simulink model "pneumaticmodelwithpressuredynamic"  (R2013a)
settings: Solver=ode4  StartTime=0.0  StopTime=20  FixedStep=0.005  RelTol=1e-3
libraries: simulink x5, cstblocks x5
settings Model: Creator=gkharish  LastModifiedBy=gkharish

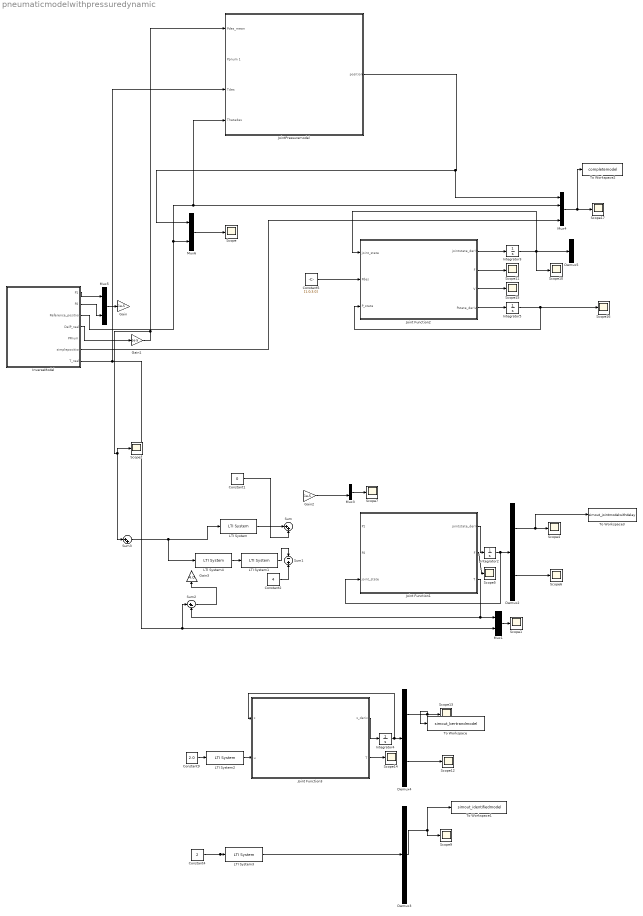
== system pneumaticmodelwithpressuredynamic ==
  Constant1 : Constant  Value=0
  Constant2 : Constant  Value=4
  Constant4 : Constant  Value=2
  Constant5 : Constant  Value=[1.0;3.0]
  Constant9 : Constant  Value=2.0
  Demux2 : Demux  Outputs=2
  Demux3 : Demux  Outputs=1
  Demux4 : Demux  Outputs=2
  Demux5 : Demux  Outputs=2
  Gain : Gain  Gain=1e-5
  Gain1 : Gain  Gain=1e-5
  Gain2 : Gain  Gain=1e-5
  Gain3 : Gain  Gain=4.0
  Integrator2 : Integrator  InitialCondition=[0 0]
  Integrator3 : Integrator  InitialCondition=[0 0]
  Integrator4 : Integrator  InitialCondition=[0 0]
  Integrator5 : Integrator  InitialCondition=[0 0 4 0]
  InverseModel : Subsystem
  Joint Function1 : MATLAB Function  TreatAsAtomicUnit=on
  Joint Function2 : MATLAB Function  TreatAsAtomicUnit=on
  Joint Function3 : MATLAB Function  TreatAsAtomicUnit=on
  "JointPressuremodel " : Subsystem
  LTI System : cstblocks/LTI System  sys=tf(1, [0.17 1])  IC=[]
  LTI System1 : cstblocks/LTI System  sys=tf(1, [0.5 1])  IC=[]
  LTI System2 : cstblocks/LTI System  sys=tf(1, [0.2 1])  IC=[]
  LTI System3 : cstblocks/LTI System  sys=tf(1, [0.17 1])  IC=[]
  LTI System4 : cstblocks/LTI System  sys=tf(1, [0.5 1])  IC=[]
  Mux1 : Mux  Inputs=2
  Mux3 : Mux  Inputs=3
  Mux4 : Mux
  Mux5 : Mux  Inputs=2
  Mux6 : Mux  Inputs=2
  Scope{,1..2,4..7,9..17} (16 alike) : Scope
      Scope settings: SaveName=ScopeData19
      Scope1 settings: ShowLegends=on  SaveName=ScopeData26
      Scope10 settings: SaveName=ScopeData9
      Scope11 settings: SaveName=ScopeData11
      Scope12 settings: SaveName=ScopeData12
      Scope13 settings: ShowLegends=on  SaveName=ScopeData13
      Scope14 settings: ShowLegends=on  SaveName=ScopeData14
      Scope15 settings: ShowLegends=on  SaveName=ScopeData15
      Scope16 settings: SaveName=ScopeData16
      Scope17 settings: ShowLegends=on  YMin=-0.8  YMax=0.9  SaveName=ScopeData17
      Scope2 settings: ShowLegends=on  SaveName=ScopeData28
      Scope4 settings: ShowLegends=on  SaveName=ScopeData4
      Scope5 settings: ShowLegends=on  SaveName=ScopeData5
      Scope6 settings: SaveName=ScopeData6
      Scope7 settings: ShowLegends=on  SaveName=ScopeData7
      Scope9 settings: ShowLegends=on  SaveName=ScopeData10
  Sum : Sum  Inputs=|++
  Sum1 : Sum  Inputs=-+
  Sum2 : Sum  Inputs=|+-
  Sum3 : Sum  Inputs=|++
  To Workspace : ToWorkspace  VariableName=simout_bertrandmodel  SampleTime=-1  SaveFormat=Timeseries
  To Workspace1 : ToWorkspace  VariableName=simout_identifiedmodel  SampleTime=-1  SaveFormat=Timeseries
  To Workspace2 : ToWorkspace  VariableName=completemodel  SampleTime=-1  SaveFormat=Timeseries
  To Workspace3 : ToWorkspace  VariableName=simout_jointmodelwithdelay  SampleTime=-1  SaveFormat=Timeseries
  wires:
  Joint Function1/1(jointstate_deriv) -> Integrator2/1
  Integrator2/1 -> Demux2/1, Joint Function1/3(joint_state)
  Demux2/1 -> To Workspace3/1, Scope4/1
  Joint Function1/2(F) -> Scope5/1
  Demux2/2 -> Scope6/1
  Mux3/1 -> Scope7/1
  InverseModel/4(DelP_real) -> Gain1/1
  Joint Function3/1(x_deriv) -> Integrator4/1
  Integrator4/1 -> Joint Function3/1(x), Demux4/1
  Demux4/1 -> To Workspace/1, Scope13/1
  Demux4/2 -> Scope12/1
  Joint Function3/2(T) -> Scope14/1
  Demux3/1 -> Scope9/1, To Workspace1/1
  LTI System3/1 -> Demux3/1
  Constant4/1 -> LTI System3/1
  Joint Function2/1(jointstate_deriv) -> Integrator3/1
  Joint Function2/4(Pstate_deriv) -> Integrator5/1
  Integrator3/1 -> Scope10/1, Demux5/1, Joint Function2/1(joint_state)
  Joint Function2/2(F) -> Scope11/1
  Joint Function2/3(V) -> Scope15/1
  Integrator5/1 -> Joint Function2/3(P_state), Scope16/1
  Constant5/1 -> Joint Function2/2(Pdes)
  Mux4/1 -> To Workspace2/1, Scope17/1
  Constant9/1 -> LTI System2/1
  LTI System2/1 -> Joint Function3/2(u)
  Mux6/1 -> Scope/1
  Mux5/1 -> Gain/1
  InverseModel/1(P1) -> Mux5/1
  InverseModel/2(P2) -> Mux5/2
  InverseModel/3(Reference_position) -> "JointPressuremodel "/4(Thetades), Mux4/2, Mux6/2
  "JointPressuremodel "/1(position) -> Mux4/1, Mux6/1
  InverseModel/6(simpleposition) -> Mux4/4
  Gain2/1 -> Mux3/3
  Joint Function1/3(T) -> Mux1/1, Sum2/2
  Mux1/1 -> Scope1/1
  InverseModel/7(T_real) -> "JointPressuremodel "/3(Tdes), Sum2/1, Mux1/2
  Sum2/1 -> Gain3/1
  Gain1/1 -> "JointPressuremodel "/1("Pdes_mean "), Scope2/1, Sum3/1
  Sum3/1 -> LTI System/1, LTI System4/1
  Constant2/1 -> Sum1/2
  LTI System1/1 -> Sum1/1
  LTI System/1 -> Sum/1
  Constant1/1 -> Sum/2
  LTI System4/1 -> LTI System1/1
  ? -> Mux4/3

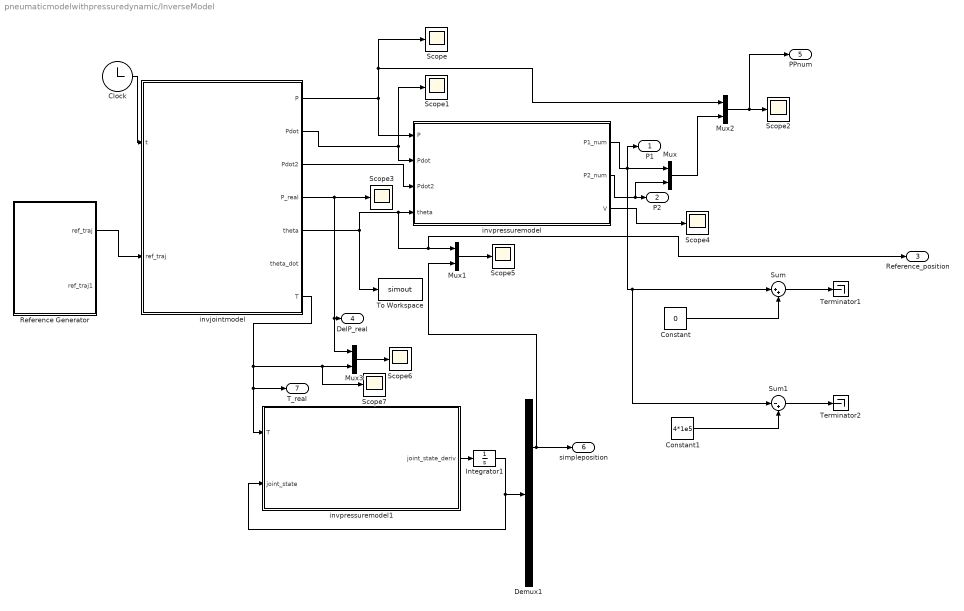
== system pneumaticmodelwithpressuredynamic/InverseModel ==
  Clock : Clock
  Constant : Constant  Value=0
  Constant1 : Constant  Value=4*1e5
  Demux1 : Demux  Outputs=2
  Integrator1 : Integrator  InitialCondition=[0 0]
  Mux{,1..3} (4 alike) : Mux  Inputs=2
  Reference Generator : Subsystem
  Scope{,1..7} (8 alike) : Scope
      Scope settings: SaveName=ScopeData8
      Scope1 settings: SaveName=ScopeData9
      Scope2 settings: ShowLegends=on
      Scope4 settings: SaveName=ScopeData2
      Scope5 settings: ShowLegends=on  SaveName=ScopeData22
      Scope6 settings: ShowLegends=on  SaveName=ScopeData23
      Scope7 settings: ShowLegends=on  SaveName=ScopeData24
  Sum : Sum  Inputs=|++
  Sum1 : Sum  Inputs=|-+
  Terminator1 : Terminator
  Terminator2 : Terminator
  To Workspace : ToWorkspace  VariableName=simout  SampleTime=-1  SaveFormat=Timeseries
  invjointmodel : MATLAB Function  TreatAsAtomicUnit=on
  invpressuremodel : MATLAB Function  TreatAsAtomicUnit=on
  invpressuremodel1 : MATLAB Function  TreatAsAtomicUnit=on
  P1 : Outport
  P2 : Outport  Port=2
  Reference_position : Outport  Port=3
  DelP_real : Outport  Port=4
  PPnum : Outport  Port=5
  simpleposition : Outport  Port=6
  T_real : Outport  Port=7
  wires:
  invjointmodel/2(Pdot) -> invpressuremodel/2(Pdot), Scope1/1
  Clock/1 -> invjointmodel/1(t)
  invpressuremodel/1(P1_num) -> P1/1, Mux/1, Sum/1, Sum1/1
  Constant1/1 -> Sum1/2
  invjointmodel/5(theta) -> Reference_position/1, Mux1/1, invpressuremodel/4(theta), To Workspace/1
  Constant/1 -> Sum/2
  invjointmodel/1(P) -> Mux2/1, Scope/1, invpressuremodel/1(P)
  invjointmodel/3(Pdot2) -> invpressuremodel/3(Pdot2)
  Sum/1 -> Terminator1/1
  Sum1/1 -> Terminator2/1
  invpressuremodel/2(P2_num) -> P2/1, Mux/2
  invjointmodel/4(P_real) -> Mux3/1, DelP_real/1, Scope3/1
  invpressuremodel/3(V) -> Scope4/1
  Integrator1/1 -> invpressuremodel1/2(joint_state), Demux1/1
  invpressuremodel1/1(joint_state_deriv) -> Integrator1/1
  Demux1/1 -> simpleposition/1, Mux1/2
  Mux1/1 -> Scope5/1
  Mux/1 -> Mux2/2
  Mux2/1 -> PPnum/1, Scope2/1
  Mux3/1 -> Scope6/1
  invjointmodel/7(T) -> Scope7/1, Mux3/2, T_real/1, invpressuremodel1/1(T)
  Reference Generator/1(ref_traj) -> invjointmodel/2(ref_traj)

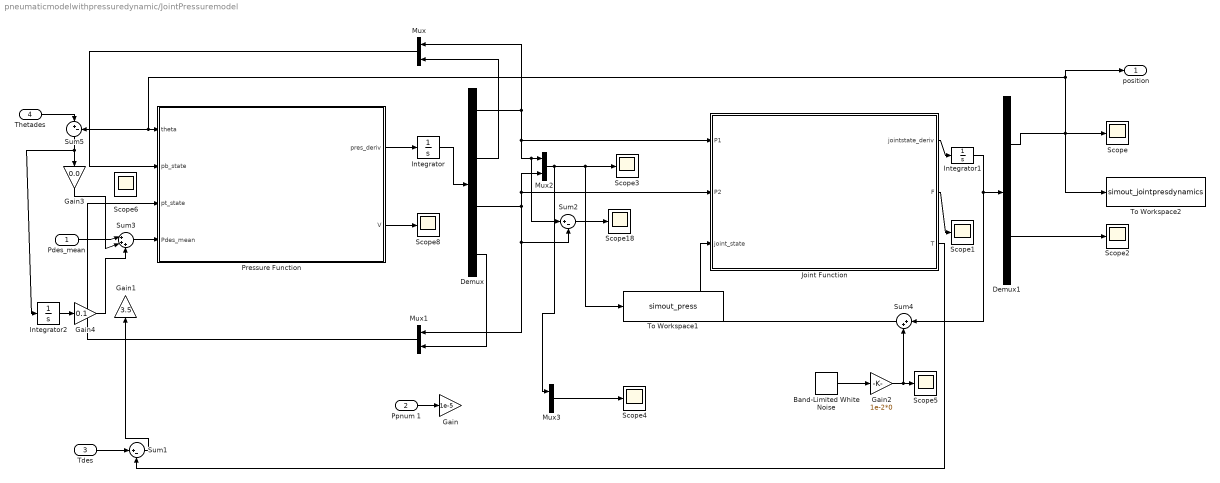
== system pneumaticmodelwithpressuredynamic/JointPressuremodel  ==
  "Pdes_mean " : Inport
  Ppnum 1 : Inport  Port=2
  Tdes : Inport  Port=3
  Thetades : Inport  Port=4
  Band-Limited White Noise : simulink/Sources/Band-Limited White Noise  Cov=[0.1]  Ts=0.005  seed=[23341]
  Demux : Demux
  Demux1 : Demux  Outputs=2
  Gain : Gain  Gain=1e-5
  Gain1 : Gain  Gain=3.5
  Gain2 : Gain  Gain=1e-2*0
  Gain3 : Gain  Gain=0.0
  Gain4 : Gain  Gain=0.1
  Integrator : Integrator  InitialCondition=[0 0 4 0]
  Integrator1 : Integrator  InitialCondition=[0 0]
  Integrator2 : Integrator
  Joint Function : MATLAB Function  TreatAsAtomicUnit=on
  Mux{,1..3} (4 alike) : Mux  Inputs=2
  Pressure Function : MATLAB Function  TreatAsAtomicUnit=on
  Scope{,1..6,8,18} (9 alike) : Scope
      Scope settings: ShowLegends=on
      Scope1 settings: ShowLegends=on  TimeRange=10  YMin=240  YMax=285
      Scope18 settings: ShowLegends=on  SaveName=ScopeData18
      Scope2 settings: SaveName=ScopeData2
      Scope3 settings: ShowLegends=on  SaveName=ScopeData3
      Scope4 settings: ShowLegends=on  SaveName=ScopeData25
      Scope5 settings: ShowLegends=on  SaveName=ScopeData27
      Scope6 settings: ShowLegends=on  SaveName=ScopeData29
      Scope8 settings: ShowLegends=on  SaveName=ScopeData8
  Sum1 : Sum  Inputs=|+-
  Sum2 : Sum  Inputs=|+-
  Sum3 : Sum  Inputs=|+++
  Sum4 : Sum  Inputs=|++
  Sum5 : Sum  Inputs=|+-
  To Workspace1 : ToWorkspace  VariableName=simout_press  SampleTime=-1  SaveFormat=Timeseries
  To Workspace2 : ToWorkspace  VariableName=simout_jointpresdynamics  SampleTime=-1  SaveFormat=Timeseries
  position : Outport
  wires:
  Demux/1 -> Sum2/1, Mux2/1, Joint Function/1(P1), Mux/1
  Integrator1/1 -> Sum4/1, Demux1/1
  Pressure Function/2(V) -> Scope8/1
  Mux1/1 -> Pressure Function/3(pt_state)
  Demux/2 -> Mux/2
  Joint Function/1(jointstate_deriv) -> Integrator1/1
  Demux/4 -> Mux1/2
  Demux1/2 -> Scope2/1
  Demux1/1 -> To Workspace2/1, Sum5/2, Pressure Function/1(theta), position/1, Scope/1
  Joint Function/2(F) -> Scope1/1
  Pressure Function/1(pres_deriv) -> Integrator/1
  Mux/1 -> Pressure Function/2(pb_state)
  Integrator/1 -> Demux/1
  Sum2/1 -> Scope18/1
  Demux/3 -> Sum2/2, Mux1/1, Mux2/2, Joint Function/2(P2)
  Mux3/1 -> Scope4/1
  Ppnum 1/1 -> Gain/1
  "Pdes_mean "/1 -> Sum3/1
  Sum3/1 -> Pressure Function/4(Pdes_mean)
  Sum1/1 -> Gain1/1
  Mux2/1 -> Mux3/1, To Workspace1/1, Scope3/1
  Joint Function/3(T) -> Sum1/2
  Band-Limited White Noise/1 -> Gain2/1
  Sum4/1 -> Joint Function/3(joint_state)
  Gain2/1 -> Sum4/2, Scope5/1
  Tdes/1 -> Sum1/1
  Thetades/1 -> Sum5/1
  Sum5/1 -> Integrator2/1, Gain3/1
  Integrator2/1 -> Gain4/1
  Gain4/1 -> Sum3/3
  Gain3/1 -> Sum3/2

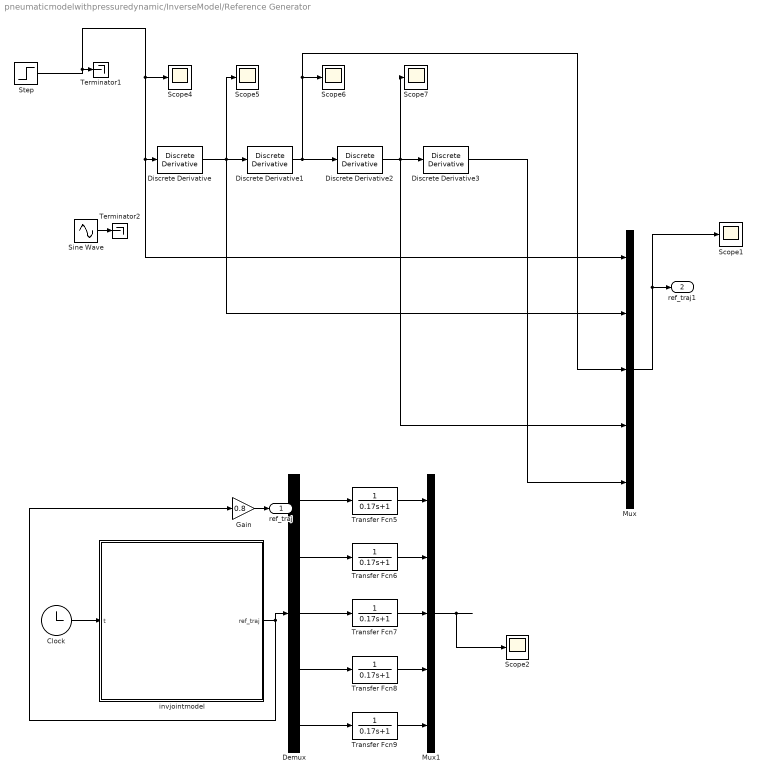
== system pneumaticmodelwithpressuredynamic/InverseModel/Reference Generator ==
  Clock : Clock
  Demux : Demux  Outputs=5
  Discrete Derivative{,1..3} (4 alike) : simulink/Discrete/Discrete Derivative  gainval=1.0  ICPrevScaledInput=0.0  InputProcessing=Inherited  OutMin=[]  OutMax=[]  OutDataType=fixdt(1, 16)  OutScaling=2^-10  DoSatur=off
  Gain : Gain  Gain=0.8
  Mux : Mux  Inputs=5
  Mux1 : Mux  Inputs=5
  Scope{1..2,4..7} (6 alike) : Scope
      Scope1 settings: ShowLegends=on  SaveName=ScopeData20
      Scope2 settings: ShowLegends=on  SaveName=ScopeData21
      Scope4 settings: SaveName=ScopeData4
      Scope5 settings: SaveName=ScopeData5
      Scope6 settings: SaveName=ScopeData6
      Scope7 settings: SaveName=ScopeData7
  Sine Wave : Sin  Amplitude=1.0  SampleTime=0
  Step : Step  SampleTime=0
  Terminator1 : Terminator
  Terminator2 : Terminator
  Transfer Fcn{5..9} (5 alike) : TransferFcn  Denominator=[0.17 1]
  invjointmodel : MATLAB Function  TreatAsAtomicUnit=on
  ref_traj : Outport
  ref_traj1 : Outport  Port=2
  wires:
  Mux/1 -> ref_traj1/1, Scope1/1
  Step/1 -> Mux/1, Discrete Derivative/1, Scope4/1, Terminator1/1
  Discrete Derivative/1 -> Mux/2, Scope5/1, Discrete Derivative1/1
  Discrete Derivative1/1 -> Mux/3, Scope6/1, Discrete Derivative2/1
  Discrete Derivative2/1 -> Mux/4, Discrete Derivative3/1, Scope7/1
  Discrete Derivative3/1 -> Mux/5
  Clock/1 -> invjointmodel/1(t)
  invjointmodel/1(ref_traj) -> Demux/1, Gain/1
  Transfer Fcn5/1 -> Mux1/1
  Transfer Fcn6/1 -> Mux1/2
  Transfer Fcn7/1 -> Mux1/3
  Transfer Fcn8/1 -> Mux1/4
  Transfer Fcn9/1 -> Mux1/5
  Demux/1 -> Transfer Fcn5/1
  Demux/4 -> Transfer Fcn8/1
  Demux/5 -> Transfer Fcn9/1
  Demux/3 -> Transfer Fcn7/1
  Demux/2 -> Transfer Fcn6/1
  Mux1/1 -> Scope2/1
  Gain/1 -> ref_traj/1
  Sine Wave/1 -> Terminator2/1

== matlab function pneumaticmodelwithpressuredynamic/JointPressuremodel /Joint Function ==
  data: P1 input; jointstate_deriv output; P2 input; joint_state input; F output; T output
function [jointstate_deriv,F, T] = jointdynamics(P1, P2, joint_state)
jointstate_deriv = zeros(2,1);
theta = joint_state(1);
theta_dot = joint_state(2);
%% Parameters for the muscles
lo = 0.185;
alphao = 23.0*pi/180;
%epsilono = 0.15;
%emax = 0.2983;
k = 1.25;
ro = 0.009;
R = 0.015;

a = 3/(tan(alphao))^2;
b = 1/(sin(alphao))^2;
emax = (1/k)*(1 - sqrt(b/a));

lb = lo- R*theta;
epsb = (1-(lb/lo));
lt = lo*(1-emax) + R*theta;
epst = (1-(lt/lo));

%% Parameters of Joint
m = 2.6;
link_l = 0.32;
g =9.81;
I = m*(link_l^2)/3;
fv = 0.25;


F1 =  pi*ro^2*P1*1e5*(a*(1-k*epsb)^2 - b);
F2 =  pi*ro^2*P2*1e5*(a*(1-k*epst)^2 - b);
F2max = 1*pi*ro^2*4*1e5*(a*(1-k*emax)^2 - b);
T = (F1 -F2 )*R;
F = [F1 F2 T];
jointstate_deriv(1) = theta_dot; %joint_state(2);
jointstate_deriv(2) = ((F1 -F2 )*R  - fv*theta_dot - m*g*0.5*link_l*sin(theta))/I;

== matlab function pneumaticmodelwithpressuredynamic/JointPressuremodel /Pressure Function ==
  data: theta input; pres_deriv output; pb_state input; pt_state input; Pdes_mean input; V output
function [pres_deriv,V] = pressuredynamics(theta, pb_state, pt_state, Pdes_mean)

pres_deriv = zeros(4,1);
V = zeros(2,1);
Pdes = zeros(2,1);
%% Parameters for the muscles
lo = 0.185;
alphao = 23.0*pi/180;
%epsilono = 0.15;
%emax = 0.2983;
k = 1.25;
ro = 0.009;
R = 0.015;
a = 3/(tan(alphao))^2;
b = 1/(sin(alphao))^2;
emax = (1/k)*(1 - sqrt(b/a));
%% Calculate Volume 
% biceps agonistic muscle
lb = lo - R*theta;
cs2 = (cos(alphao))^2;
epsb2 = (1-(lb/lo))^2;
termb1 = (1 - cs2*epsb2);

Vb = 1e6*(pi*lb*ro^2/((sin(alphao))^2))*termb1
%Vb = 230;
wnb = 2*pi*380*(1/Vb)

% triceps antagonistic muscle 
lt = lo*(1-emax) + R*theta; 
cs2 = (cos(alphao))^2;
epst2 = (1-(lt/lo))^2;
termt1 = (1 - cs2*epst2);

Vt = 1e6*(pi*lt*ro^2/((sin(alphao))^2))*termt1
%Vt = 230;
wnt = 2*pi*380*(1/Vt)

Pdes(1) = Pdes_mean;
Pdes(2) = 4 - Pdes_mean;

pres_deriv(1) = pb_state(2);
pres_deriv(2) = -wnb^2*pb_state(1) - 2*wnb*1*pb_state(2) + (wnb^2)*Pdes(1);

pres_deriv(3) = pt_state(2);
pres_deriv(4) = -wnt^2*pt_state(1) - 2*wnt*1*pt_state(2) + (wnt^2)*Pdes(2);

% pres_deriv(5) = Vb;
% pres_deriv(6) = Vt;
V = [Vb;Vt];

== matlab function pneumaticmodelwithpressuredynamic/Joint Function1 ==
  data: P1 input; jointstate_deriv output; P2 input; joint_state input; F output; T output
function [jointstate_deriv,F,T] = jointdynamics(P1, P2, joint_state)
jointstate_deriv = zeros(2,1);
theta = joint_state(1);
theta_dot = joint_state(2);
%% Parameters for the muscles
lo = 0.185;
alphao = 23.0*pi/180;
%epsilono = 0.15;
%emax = 0.2983;
k = 1.25;
ro = 0.009;
R = 0.015;

a = 3/(tan(alphao))^2;
b = 1/(sin(alphao))^2;
emax = (1/k)*(1 - sqrt(b/a));

lb = lo- R*theta;
epsb = (1-(lb/lo));
lt = lo*(1-emax) + R*theta;
epst = (1-(lt/lo));

%% Parameters of Joint
m = 2.6;
link_l = 0.32;
g =9.81;
I = m*(link_l^2)/3;
fv = 0.25;


F1 =  pi*ro^2*P1*1e5*(a*(1-k*epsb)^2 - b);
F2 =  pi*ro^2*P2*1e5*(a*(1-k*epst)^2 - b);
F2max = 1*pi*ro^2*4*1e5*(a*(1-k*emax)^2 - b);
F = [F1 F2];
jointstate_deriv(1) = theta_dot; %joint_state(2);
jointstate_deriv(2) = ((F1 -F2 )*R  - fv*theta_dot - m*g*0.5*link_l*sin(theta))/I;
T = (F1 -F2 )*R ;

== matlab function pneumaticmodelwithpressuredynamic/Joint Function2 ==
  data: joint_state input; Pdes input; P_state input; jointstate_deriv output; F output; V output; Pstate_deriv output
function [jointstate_deriv,F,V,Pstate_deriv] = jointpressuredynamics(joint_state, Pdes, P_state)
jointstate_deriv = zeros(2,1);
F = zeros(2,1);
V = zeros(2,1);
Pstate_deriv = zeros(4,1);
theta = joint_state(1);
theta_dot = joint_state(2);
%% Parameters for the muscles
lo = 0.185;
alphaob = 23.0*pi/180;
alphaot = 23.0*pi/180;
k = 1.25;
ro = 0.009;
R = 0.015;

a_biceps = 3/(tan(alphaob))^2;
b_biceps = 1/(sin(alphaob))^2;
emax_biceps = (1/k)*(1 - sqrt(b_biceps/a_biceps));

a_triceps = 3/(tan(alphaot))^2;
b_triceps = 1/(sin(alphaot))^2;
emax_triceps = (1/k)*(1 - sqrt(b_triceps/a_triceps));

lb = lo- R*theta;
epsb = (1-(lb/lo));
lt = lo*(1-emax_triceps) + R*theta;
epst = (1-(lt/lo));

%% Parameters of Joint
m = 2.6;
link_l = 0.32;
g =9.81;
I = m*(link_l^2)/3;
fv = 0.25;
%% Volume calcuation
% biceps agonistic muscle
lb = lo - R*theta;
csb2 = (cos(alphaob))^2;
epsb2 = (1-(lb/lo))^2;
termb1 = (1 - csb2*epsb2);

Vb = 1e6*(pi*lb*ro^2/((sin(alphaob))^2))*termb1
%Vb = 1630;
wnb = 2*pi*380*(1/Vb)

% triceps antagonistic muscle 
lt = lo*(1-emax_triceps) + R*theta; 
cst2 = (cos(alphaot))^2;
epst2 = (1-(lt/lo))^2;
termt1 = (1 - cst2*epst2);

Vt = 1e6*(pi*lt*ro^2/((sin(alphaot))^2))*termt1
%Vt = 1630;
wnt = 2*pi*380*(1/Vt)

V = [Vb;Vt];

%% Pressure Dynamics
Pb_state = P_state(1:2,1);
Pt_state = P_state(3:4,1);
Pstate_deriv(1) = Pb_state(2);
Pstate_deriv(2) = -wnb^2*Pb_state(1) - 2*wnb*1*Pb_state(2) + (wnb^2)*Pdes(1);

Pstate_deriv(3) = Pt_state(2);
Pstate_deriv(4) = -wnt^2*Pt_state(1) - 2*wnt*1*Pt_state(2) + (wnt^2)*Pdes(2);

%% Force calculation
P1 = Pb_state(1);
P2 = Pt_state(1);
F_biceps =  pi*ro^2*P1*1e5*(a_biceps*(1-k*epsb)^2 - b_biceps);
F_triceps =  pi*ro^2*P2*1e5*(a_triceps*(1-k*epst)^2 - b_triceps);
%F2max = 1*pi*ro^2*4*1e5*(a*(1-k*emax)^2 - b);
F = [F_biceps; F_triceps];

%% Joint Dynamics
jointstate_deriv(1) = theta_dot; %joint_state(2);
jointstate_deriv(2) = ((F_biceps -F_triceps )*R  - fv*theta_dot - m*g*0.5*link_l*sin(theta))/I;


%% END

== matlab function pneumaticmodelwithpressuredynamic/Joint Function3 ==
  data: x input; x_deriv output; u input; T output
function [x_deriv,T] = bertrand_system(x, u)


%[row col] = size(x);
x_deriv = zeros(size(x));
theta = x(1);

% g = 9.8;
% m = 2.75;
% link_l = 0.32;
% 
% I = m*(link_l^2)/3;
% K1 = 2.1794;
% K2 = 1.2698;
% Pm = 2.5 ;
% 
% Tmax = 5*K1;
% fk = 0.1*Tmax;
% fs = fk/10;
% fv = fk;
%% Parameters for the muscles
lo = 0.185;
alphaob = 23.0*pi/180;
alphaot = 23.0*pi/180;
k = 1.25;
ro = 0.009;
R = 0.015;

a_biceps = 3/(tan(alphaob))^2;
b_biceps = 1/(sin(alphaob))^2;
emax_biceps = (1/k)*(1 - sqrt(b_biceps/a_biceps));

a_triceps = 3/(tan(alphaot))^2;
b_triceps = 1/(sin(alphaot))^2;
emax_triceps = (1/k)*(1 - sqrt(b_triceps/a_triceps));

lb = lo- R*theta;
epsb = (1-(lb/lo));
lt = lo*(1-emax_triceps) + R*theta;
epst = (1-(lt/lo));
%etot = 
%% Paramters of the dynamical equations
% Ko K1 K2;
Pob = 0.0; Pot = 4.0;
% Assuming that both the musclea are identical

t1 = Pob*(1 -2*k*epsb);
t2 = Pot*(1 -2*k*epst);
Ko = a_biceps*(t1 -t2) - b_biceps*(Pob - Pot);
t3 = a_biceps*(1 - k*(epsb + epst));
K1 = 2*(t3 - b_biceps);
K2 = 2*a_biceps*k*R*(Pob + Pot)/lo;

%% Parameters of Joint
m = 2.6;
link_l = 0.32;
g =9.81;
I = m*(link_l^2)/3;
fv = 0.25;

%% state equaition
x_deriv(1) = x(2);
%x_deriv(2) =  ( ( -2*K2*Pm*x(1) - m*g*(link_l/2)*sin(x(1)) -fv*x(2) + 2*K1*u ))/I;
x_deriv(2) = ((pi*ro^2*1e5)*R*(Ko + K1*u - K2*x(1)) - m*g*(link_l/2)*sin(x(1)) -fv*x(2))/I;

T = I*x_deriv(2);

== matlab function pneumaticmodelwithpressuredynamic/InverseModel/invjointmodel ==
  data: P output; Pdot output; Pdot2 output; P_real output; theta output; theta_dot output; t input; ref_traj input; T output
function [P, Pdot, Pdot2, P_real,theta, theta_dot, T] =   invjointmodel(t, ref_traj)

%% Parameters for the muscles
lo = 0.185;
alphaob = 23.0*pi/180;
alphaot = 23.0*pi/180;
k = 1.25;
ro = 0.009;
R = 0.015;

a = 3/(tan(alphaob))^2;
b = 1/(sin(alphaob))^2;
emax = (1/k)*(1 - sqrt(b/a));
Pmax = 4.0*1e5;
P1o = 0;
P2o = Pmax;
%% Parameters of Joint
m = 2.6;
link_l = 0.32;
g =9.81;
I = m*(link_l^2)/3;
fv = 0.25;

Fmax = (pi*ro^2)*(a-b)*Pmax;

%% Reference trajectory
% if(t<=5)
%     theta = 20*pi/180;
%     theta_dot = 0;
%     t1 = R*theta/(lo*emax);
%     t2 = (m*g*link_l*0.5*sin(theta))/(R*Fmax);
%     P_real = Pmax*(t1 + t2);
%     
%    
%     
%     t2dot = (m*g*link_l*0.5*cos(theta))/(R*Fmax);
%     
%     P_real_dot = Pmax*(t2dot);
% 
%     
%     t2dot2 = (- m*g*link_l*0.5*sin(theta))/(R*Fmax);
% 
%     P_real_dot2 = Pmax*(t2dot2);
% 
%     P1 = P1o + P_real;  
%     P2 = P2o - P_real;
%     
%     P1dot = P1o + P_real_dot;
%     P2dot = P2o - P_real_dot;
% 
%     P1dot2 = P1o + P_real_dot2;
%     P2dot2 = P2o - P_real_dot2;
% 
%     P = [P1 P2];
%     Pdot = [P1dot P2dot];   
%     Pdot2 = [P1dot2 P2dot2];
% %     P = [1.0 3.0];
% %     Pdot = [0 0];
% %     Pdot2 = [0 0];
%else
theta = ref_traj(1);%(t-1)*5*pi/180;         %ref_traj(1);
theta_dot = ref_traj(2);%5*pi/180;     %ref_traj(2);
theta_dot2 = ref_traj(3);
theta_dot3 = ref_traj(4);
theta_dot4 = ref_traj(5);
t1 = R*theta/(lo*emax);
t2 = (I*theta_dot2 + fv*theta_dot + m*g*link_l*0.5*sin(theta))/(R*Fmax);

P_real = Pmax*(t1 + t2);

t1dot = R*theta_dot/(lo*emax);
t2dot = (I*theta_dot3 + fv*theta_dot2 + m*g*link_l*0.5*cos(theta))/(R*Fmax);

P_real_dot = Pmax*(t1dot + t2dot);

t1dot2 = R*theta_dot2/(lo*emax);
t2dot2 = (I*theta_dot4 + fv*theta_dot3 - m*g*link_l*0.5*sin(theta))/(R*Fmax);

P_real_dot2 = Pmax*(t1dot2 + t2dot2);

P1 = P1o + P_real;
P2 = P2o - P_real;

P1dot = P_real_dot;
P2dot = -P_real_dot;

P1dot2 = P_real_dot2;
P2dot2 = -P_real_dot2;

P = [P1 P2];
Pdot = [P1dot P2dot];
Pdot2 = [P1dot2 P2dot2];

tor1 = P_real/Pmax;
tor2 = R*theta/(lo*emax);
T = R*Fmax*(tor1 -tor2);
end

== matlab function pneumaticmodelwithpressuredynamic/InverseModel/invpressuremodel ==
  data: P input; P1_num output; Pdot input; Pdot2 input; theta input; P2_num output; V output
function [P1_num, P2_num, V] = invpressuredynamic(P, Pdot, Pdot2, theta)

%% Parameters for the muscles
lo = 0.185;
alphaob = 23.0*pi/180;
alphaot = 23.0*pi/180;
k = 1.25;
ro = 0.009;
R = 0.015;

a = 3/(tan(alphaob))^2;
b = 1/(sin(alphaob))^2;
emax = (1/k)*(1 - sqrt(b/a));
Pmax = 4.0*1e5;
P1o = 0;
P2o = Pmax;
%% Parameters of Joint
m = 2.6;
link_l = 0.32;
g =9.81;
I = m*(link_l^2)/3;
fv = 0.25;

Fmax = (pi*ro^2)*(a-b)*Pmax;

%% Calculate Volume 
% biceps agonistic muscle
lb = lo - R*theta;
cs2 = (cos(alphaob))^2;
epsb2 = (1-(lb/lo))^2;
termb1 = (1 - cs2*epsb2);

Vb = 1e6*(pi*lb*ro^2/((sin(alphaob))^2))*termb1;
%Vb = 230;
wnb = 2*pi*380*(1/Vb);

% triceps antagonistic muscle 
lt = lo*(1-emax) + R*theta; 
cs2 = (cos(alphaot))^2;
epst2 = (1-(lt/lo))^2;
termt1 = (1 - cs2*epst2);

Vt = 1e6*(pi*lt*ro^2/((sin(alphaot))^2))*termt1;
%Vt = 230;
wnt = 2*pi*380*(1/Vt);

V = [Vb Vt];
%% Pressure dynamic
P1_num = P(1);% + 2*Pdot(1)/wnb + Pdot2(1)/(wnb^2);

P2_num = P(2);%  + 2*Pdot(2)/wnt + Pdot2(2)/(wnt^2);
% DelP_num = (P1_num - P2_num) + (P2o - P1o)/2;
% tor1 = DelP_num/Pmax;
% tor2 = R*theta/(lo*emax);
% Tnum = R*Fmax*(tor1 -tor2);

== matlab function pneumaticmodelwithpressuredynamic/InverseModel/Reference Generator/invjointmodel ==
  data: t input; ref_traj output
function ref_traj =   invjointmodel(t)
ref_traj = zeros(5,1);

%sine wave trajectory
f = 0.1;
a = 30*pi/180;
b = 20*pi/180;
ref_traj(1) =  a+ b*sin(2*pi*f*t);
ref_traj(2) = b*2*pi*f*cos(2*pi*f*t);
ref_traj(3) = -b*((2*pi*f)^2)*sin(2*pi*f*t);
ref_traj(4) = -b*((2*pi*f)^3)*cos(2*pi*f*t);
ref_traj(5) = b*((2*pi*f)^4)*sin(2*pi*f*t);

% %line trajectory
% ref_final = 45*pi/180;
% if (t <=3)
% ref_traj(1) = t*15*pi/180;
% ref_traj(2) = 15*pi/180;
% ref_traj(3) = 0;
% ref_traj(4) = 0;
% ref_traj(5) = 0;
% else
%     ref_traj = [ref_final 0 0 0 0]';
% end

== matlab function pneumaticmodelwithpressuredynamic/InverseModel/invpressuremodel1 ==
  data: T input; joint_state_deriv output; joint_state input
function joint_state_deriv = simplejointdynamic(T, joint_state)
joint_state_deriv = zeros(2,1);
%% Parameters for the muscles
lo = 0.185;
alphaob = 23.0*pi/180;
alphaot = 23.0*pi/180;
k = 1.25;
ro = 0.009;
R = 0.015;

a = 3/(tan(alphaob))^2;
b = 1/(sin(alphaob))^2;
emax = (1/k)*(1 - sqrt(b/a));
Pmax = 4.0*1e5;
%% Parameters of Joint
m = 2.6;
link_l = 0.32;
g =9.81;
I = m*(link_l^2)/3;
fv = 0.25;

Fmax = (pi*ro^2)*(a-b)*Pmax;


joint_state_deriv(1) = joint_state(2);
joint_state_deriv(2) = (T - fv*joint_state(2) -m*g*link_l*0.5*sin(joint_state(1)))/I;
